simulink model "rc_barometer_sim"  (R2017a)
settings: Solver=FixedStepAuto  StartTime=0.0  StopTime=30.0  RelTol=1e-3  EnableMultiTasking=on
settings Model: SimulationMode=external  Creator=Parker  LastModifiedBy=Parker
settings SolverCC: PositivePriorityOrder=on
settings OptimizationCC: PassReuseOutputArgsAs=Individual arguments  MaxStackSize=64
settings DebuggingCC: ParameterTunabilityLossMsg=error
settings HardwareCC: ProdBitPerPointer=32  ProdBitPerSizeT=32  ProdBitPerPtrDiffT=32  ProdLargestAtomicInteger=Long  ProdLargestAtomicFloat=Double  ProdWordSize=32  ProdHWDeviceType=ARM Compatible->ARM Cortex
settings SFSimCC: MATLABDynamicMemAlloc=off
settings RTWCC: SystemTargetFile=ert.tlc  HardwareBoard=Raspberry Pi  TLCOptions="-aInlineSetEventsForThisBaseRateFcn=TLC_FALSE -aSuppressMultiTaskScheduler=TLC_FALSE  -aRateBasedStepFcn=0"  TemplateMakefile=ert_default_tmf  Description=Embedded Coder  GenerateReport=on  Toolchain=GNU GCC Raspberry Pi  IncludeHyperlinkInReport=on  LaunchReport=on  GenerateTraceInfo=on  GenerateTraceReport=on  GenerateTraceReportSl=on  GenerateTraceReportSf=on  GenerateTraceReportEml=on
settings CodeAppCC: ForceParamTrailComments=on  IgnoreCustomStorageClasses=off  OperatorAnnotations=on  SimulinkDataObjDesc=on  SFDataObjDesc=on  MATLABFcnDesc=on  InsertBlockDesc=on  MATLABSourceComments=on
settings ERTTargetCC: SupportVariableSizeSignals=on

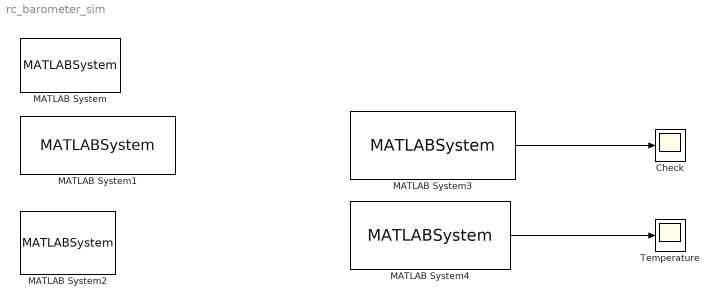
== system rc_barometer_sim ==
  Check : Scope
  MATLAB System : MATLABSystem  System=rc_initialize_sys
      mask Type: rc_initialize_sys
      mask Display: disp('rc_initialize_sys');
  MATLAB System1 : MATLABSystem  System=rc_initialize_barometer_sys
      mask Type: rc_initialize_barometer_sys
      mask Display: disp('rc_initialize_barometer_sys');
  MATLAB System2 : MATLABSystem  System=rc_cleanup_sys
      mask Type: rc_cleanup_sys
      mask Display: disp('rc_cleanup_sys');
  MATLAB System3 : MATLABSystem  System=rc_read_barometer_sys
      mask Type: rc_read_barometer_sys
      mask Display:
      | disp('rc_read_barometer_sys');
      | port_label('output',1,'y');
  MATLAB System4 : MATLABSystem  System=rc_bmp_get_temperature_sys
      mask Type: rc_bmp_get_temperature_sys
      mask Display:
      | disp('rc_bmp_get_temperature_sys');
      | port_label('output',1,'y');
  Temperature : Scope
  wires:
  MATLAB System3/1 -> Check/1
  MATLAB System4/1 -> Temperature/1
